simulink model "nl_model"  (R2024b)
settings: Solver=VariableStepAuto  StartTime=0.0  StopTime=sim.t  RelTol=1e-3
values from neighbouring files (symbols this model uses):
  params = parameters()    [lqr_main.m]    (also in sim_main.m; sim_modelling.m)
undefined symbols (not defined in the file or in its folder): cube, motor, nl_model, sim
settings Model: Creator=ben  LastModifiedBy=ben

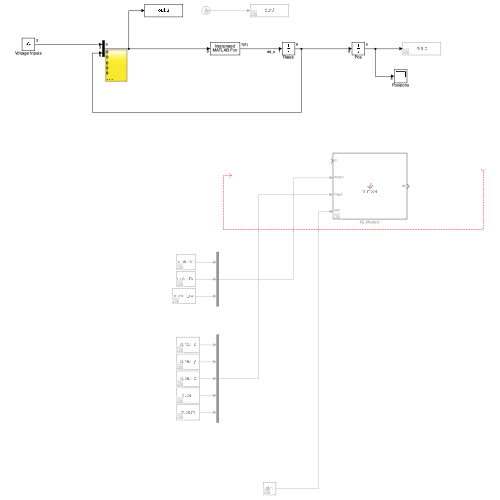
[thumbnail: Simulink's stored preview of the top-level diagram]
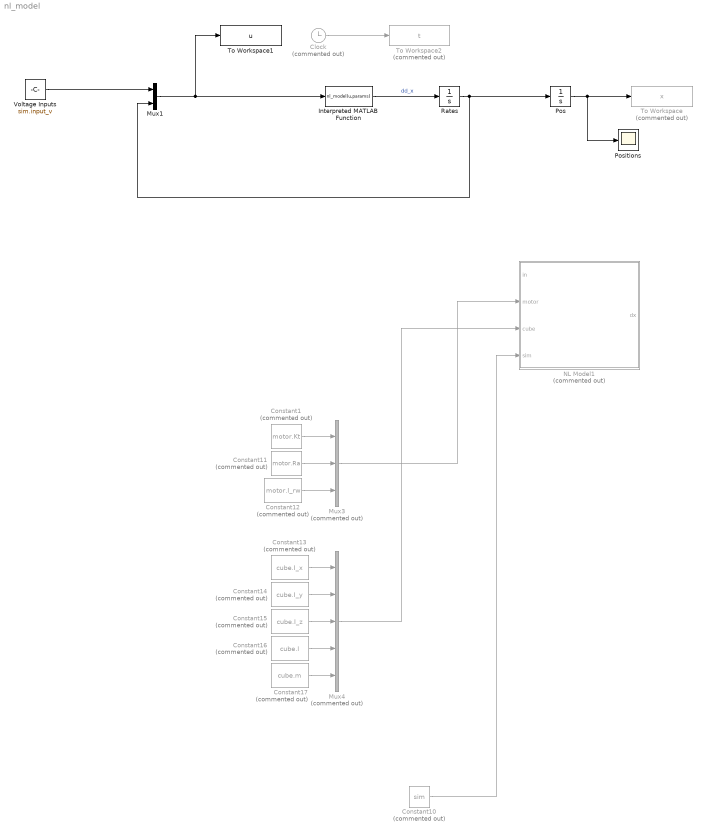
== system nl_model ==
  Clock : Clock  Commented=on
  Constant1 : Constant  Commented=on  Value=motor.Kt
  Constant10 : Constant  Commented=on  Value=sim
  Constant11 : Constant  Commented=on  Value=motor.Ra
  Constant12 : Constant  Commented=on  Value=motor.I_rw
  Constant13 : Constant  Commented=on  Value=cube.I_x
  Constant14 : Constant  Commented=on  Value=cube.I_y
  Constant15 : Constant  Commented=on  Value=cube.I_z
  Constant16 : Constant  Commented=on  Value=cube.l
  Constant17 : Constant  Commented=on  Value=cube.m
  Interpreted MATLAB Function : MATLABFcn  MATLABFcn=nl_model(u,params)  Output1D=off
  Mux1 : Mux  Inputs=2
  Mux3 : Mux  Commented=on  Inputs=3
  Mux4 : Mux  Commented=on  Inputs=5
  NL Model1 : MATLAB Function  Commented=on  TreatAsAtomicUnit=on
  Pos : Integrator  InitialCondition=sim.ic_rates
  Positions : Scope
  Rates : Integrator  InitialCondition=sim.ic_rates
  To Workspace : ToWorkspace  Commented=on  VariableName=x  SampleTime=-1
  To Workspace1 : ToWorkspace  VariableName=u  SampleTime=-1
  To Workspace2 : ToWorkspace  Commented=on  VariableName=t  SampleTime=-1
  Voltage Inputs : Constant  Value=sim.input_v
  wires:
  Mux1/1 -> To Workspace1/1, Interpreted MATLAB Function/1
  Rates/1 -> Pos/1, Mux1/2
  Interpreted MATLAB Function/1 -> Rates/1  "dd_x"
  Clock/1 -> To Workspace2/1
  Voltage Inputs/1 -> Mux1/1
  Pos/1 -> Positions/1, To Workspace/1
  ? -> ?
  Mux4/1 -> NL Model1/3(cube)
  Constant11/1 -> Mux3/2
  Mux3/1 -> NL Model1/2(motor)
  Constant10/1 -> NL Model1/4(sim)
  Constant15/1 -> Mux4/3
  Constant1/1 -> Mux3/1
  Constant17/1 -> Mux4/5
  Constant13/1 -> Mux4/1
  Constant12/1 -> Mux3/3
  Constant14/1 -> Mux4/2
  Constant16/1 -> Mux4/4

== matlab function nl_model/NL Model1 ==
  data: in input; dx output; motor input; cube input; sim input
%%% Name: Ben Miller
%%% Student Number: c3328484

function dx  = nl_model(in,motor, cube, sim)
    % State Variables
    V_a = in(1);
    V_b = in(2);
    V_c = in(3);

    alpha = in(4);
    beta = in(5);
    gamma = in(6);
    d_theta_a = in(7);
    d_theta_b = in(8);
    d_theta_c = in(9);
    

    % State Space Equations
    dd_alpha = (cube.m*sim.g*cube.l*sin(alpha)*cos(beta) - (sqrt(6)/6)*(motor.Kt/motor.Ra)*((2*V_a -V_b - V_c)-motor.Kt*(2*d_theta_a - d_theta_b - d_theta_c)))/(cube.I_y - motor.I_rw);
    dd_beta = (cube.m*sim.g*cube.l*sin(beta)*cos(alpha) - (sqrt(2)/2)*(motor.Kt/motor.Ra)*((V_b - V_c)-Kt*(d_theta_b-d_theta_c)))/(cube.I_x - motor.I_rw);
    dd_gamma = - ((sqrt(3)/3)*(motor.Kt/motor.Ra)*((V_a + V_b + V_c)-Kt*(d_theta_a + d_theta_b + d_theta_c)))/(cube.I_z - motor.I_rw);

    dd_theta_a = ((motor.Kt/motor.Ra)*(V_a - motor.Kt*d_theta_a))/(motor.I_rw);
    dd_theta_b = ((motor.Kt/motor.Ra)*(V_b - motor.Kt*d_theta_b))/(motor.I_rw);
    dd_theta_c = ((motor.Kt/motor.Ra)*(V_c - motor.Kt*d_theta_c))/(motor.I_rw);

    dx = [dd_alpha; dd_beta; dd_gamma; dd_theta_a; dd_theta_b; dd_theta_c];

end
